simulink model "comparando_simulacoes_rate_diferente_entre_sensor_e_controlador"  (R2012b)
settings: Solver=ode3  StartTime=0.0  StopTime=1  FixedStep=1e-5  RelTol=1e-6
undefined symbols (not defined in the file): J, Kd, Ke, Kt, L, P, R
libraries: simulink x86
(part 1 of 3)
settings Model: BufferReuse=off  Creator=Juliano  LastModifiedBy=Juliano
settings OptimizationCC: OptimizeBlockIOStorage=off  BufferReuse=off  ExpressionFolding=off  LocalBlockOutputs=off

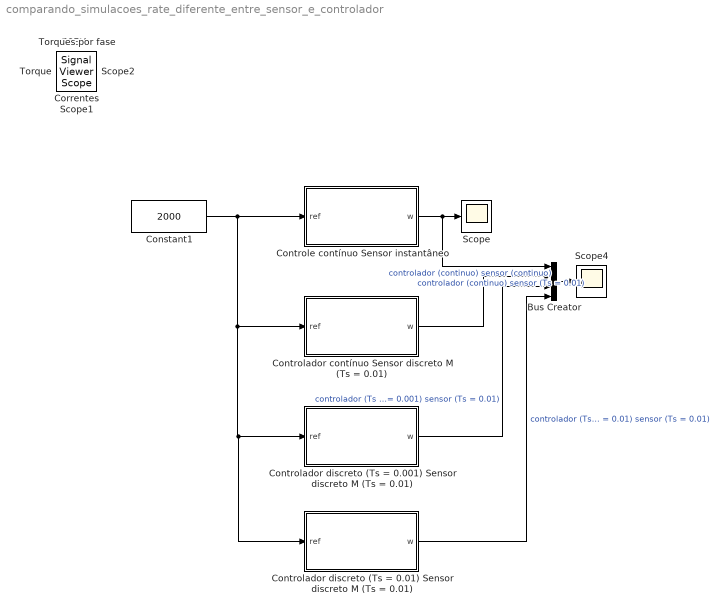
== system comparando_simulacoes_rate_diferente_entre_sensor_e_controlador ==
  Bus Creator : BusCreator
  Constant1 : Constant  Value=2000
  Controlador contínuo Sensor discreto M (Ts = 0.01) : Subsystem
  Controlador discreto (Ts = 0.001) Sensor discreto M (Ts = 0.01) : Subsystem
  Controlador discreto (Ts = 0.01) Sensor discreto M (Ts = 0.01) : Subsystem
  Controle contínuo Sensor instantâneo : Subsystem
  Scope : Scope
      settings: TimeRange=1  YMin=1600  YMax=3000
  Scope4 : Scope
      settings: ShowLegends=on  TimeRange=0.6  YMin=1100  YMax=3400  SaveName=ScopeData7
  Correntes : SignalViewerScope  IOType=viewer  NumInputPorts=3  ZoomMode=yonly  RefreshTime=0.035000
      settings: YMin=-5~-5~-5  YMax=5~5~5
  FCEMs : SignalViewerScope  IOType=viewer  NumInputPorts=3  RefreshTime=0.035000
      settings: YMin=-5~-5~-5  YMax=5~5~5  SaveName=ScopeData2
  Scope1 : SignalViewerScope  IOType=viewer  RefreshTime=0.035000
      settings: SaveName=ScopeData3
  Scope2 : SignalViewerScope  IOType=viewer  RefreshTime=0.035000
      settings: SaveName=ScopeData4
  Torque : SignalViewerScope  IOType=viewer  ZoomMode=xonly  RefreshTime=0.035000
      settings: SaveToWorkspace=on  SaveName=Torque
  Torques por fase : SignalViewerScope  IOType=viewer  NumInputPorts=3  ZoomMode=xonly  RefreshTime=0.035000
      settings: YMin=-5~-5~-5  YMax=5~5~5
  wires:
  Bus Creator/1 -> Scope4/1
  Controle contínuo Sensor instantâneo/1(w) -> Bus Creator/1, Scope/1  "controlador (continuo) sensor (continuo)"
  Constant1/1 -> Controlador contínuo Sensor discreto M (Ts = 0.01)/1(ref), Controlador discreto (Ts = 0.01) Sensor discreto M (Ts = 0.01)/1(ref), Controlador discreto (Ts = 0.001) Sensor discreto M (Ts = 0.01)/1(ref), Controle contínuo Sensor instantâneo/1(ref)
  Controlador discreto (Ts = 0.001) Sensor discreto M (Ts = 0.01)/1(w) -> Bus Creator/3  "controlador (Ts = 0.001) sensor (Ts = 0.01)"
  Controlador contínuo Sensor discreto M (Ts = 0.01)/1(w) -> Bus Creator/2  "controlador (continuo) sensor (Ts = 0.01)"
  Controlador discreto (Ts = 0.01) Sensor discreto M (Ts = 0.01)/1(w) -> Bus Creator/4  "controlador (Ts = 0.01) sensor (Ts = 0.01)"

== system comparando_simulacoes_rate_diferente_entre_sensor_e_controlador/Controlador contínuo Sensor discreto M (Ts = 0.01) ==
  ref : Inport
  Add2 : Sum  Inputs=-+|
  Anti-horário1 : Constant
  BLDC1 : Subsystem
  "Conversao deg/s -> rad/s" : Gain  Gain=pi/180
  Conversao rad-> deg : Gain  Gain=180/pi
  "Conversao rad/s -> RPM1" : Gain  Gain=60/(2*pi)
  "Conversao rad/s -> rpm" : Gain  Gain=60/(2*pi)
  Decoder1 : Subsystem
  Encoder : Subsystem  mask{Nr=360}
      mask prompts: Nr "Número de pulsos por revolução"
  Gain1 : Gain  Gain=P/2
  Inversor1 : Subsystem
  PID Controller1 : simulink/Continuous/PID Controller  Controller=PI  TimeDomain=Continuous-time  SampleTime=1  IntegratorMethod=Forward Euler  FilterMethod=Forward Euler  Form=Parallel  P=0.000518154594293452  I=0.0431725782178291  D=0  N=100  InitialConditionSource=internal  InitialConditionForIntegrator=0  InitialConditionForFilter=0  ExternalReset=none  ZeroCross=off  LimitOutput=on  UpperSaturationLimit=12  LowerSaturationLimit=-12  LinearizeAsGain=off  AntiWindupMode=none  Kb=1  TrackingMode=off  Kt=1  PParamMin=[ ]  PParamMax=[ ]  IParamMin=[ ]  IParamMax=[ ]  DParamMin=[ ]  DParamMax=[ ]  NParamMin=[ ]  NParamMax=[ ]  KbParamMin=[ ]  KbParamMax=[ ]  KtParamMin=[ ]  KtParamMax=[ ]  POutMin=[ ]  POutMax=[ ]  IOutMin=[ ]  IOutMax=[ ]  DOutMin=[ ]  DOutMax=[ ]  NOutMin=[ ]  NOutMax=[ ]  KbOutMin=[ ]  KbOutMax=[ ]  KtOutMin=[ ]  KtOutMax=[ ]  IntegratorOutMin=[ ]  IntegratorOutMax=[ ]  FilterOutMin=[ ]  FilterOutMax=[ ]  SumOutMin=[ ]  SumOutMax=[ ]  SumI1OutMin=[ ]  SumI1OutMax=[ ]  SumI2OutMin=[ ]  SumI2OutMax=[ ]  SumI3OutMin=[ ]  SumI3OutMax=[ ]  SumDOutMin=[ ]  SumDOutMax=[ ]  SaturationOutMin=[ ]  SaturationOutMax=[ ]  IntegratorContinuousStateAttributes=''  IntegratorStateMustResolveToSignalObject=off  IntegratorRTWStateStorageClass=Auto  FilterContinuousStateAttributes=''  FilterStateMustResolveToSignalObject=off  FilterRTWStateStorageClass=Auto
  Sensores Hall1 : Subsystem  AncestorBlock=spsPMSynchronousMachineModel/Discrete Trapezoidal/Hall effect sensor
  Step1 : Step  Time=0.2  After=0*2e-3  SampleTime=0
  w : Outport
  wires:
  Conversao rad-> deg/1 -> Encoder/1(Theta)
  "Conversao deg/s -> rad/s"/1 -> "Conversao rad/s -> rpm"/1
  ref/1 -> Add2/2
  PID Controller1/1 -> Inversor1/2(Vcc)
  "Conversao rad/s -> RPM1"/1 -> w/1
  Sensores Hall1/1(Hall) -> Decoder1/1("Hall ")
  Anti-horário1/1 -> Decoder1/2(Sentido de rotação)
  Inversor1/2(Vb) -> BLDC1/2(Vb)
  Add2/1 -> PID Controller1/1
  Inversor1/1(Va) -> BLDC1/1(Va)
  Decoder1/1(Gates) -> Inversor1/1(Gates)
  Inversor1/3(Vc) -> BLDC1/3(Vc)
  Gain1/1 -> Sensores Hall1/1(teta_e)
  BLDC1/1(Theta_m) -> Conversao rad-> deg/1, Gain1/1
  BLDC1/2(w_m) -> "Conversao rad/s -> RPM1"/1
  Step1/1 -> BLDC1/4(Tl)
  Encoder/3(VelocidadeM) -> "Conversao deg/s -> rad/s"/1
  "Conversao rad/s -> rpm"/1 -> Add2/1

== system comparando_simulacoes_rate_diferente_entre_sensor_e_controlador/Controlador discreto (Ts = 0.001) Sensor discreto M (Ts = 0.01) ==
  ref : Inport
  Add2 : Sum  Inputs=-+|
  Anti-horário1 : Constant
  BLDC1 : Subsystem
  "Conversao deg/s -> rad/s" : Gain  Gain=pi/180
  Conversao rad-> deg : Gain  Gain=180/pi
  "Conversao rad/s -> RPM1" : Gain  Gain=60/(2*pi)
  "Conversao rad/s -> rpm" : Gain  Gain=60/(2*pi)
  Decoder1 : Subsystem
  Discrete Transfer Fcn : DiscreteTransferFcn  Numerator=[-0.000518155 0.000474982]  Denominator=[-1 1]  SampleTime=0.001
  Encoder : Subsystem  mask{Nr=360}
      mask prompts: Nr "Número de pulsos por revolução"
  Gain1 : Gain  Gain=P/2
  Inversor1 : Subsystem
  Rate Transition : RateTransition  OutPortSampleTimeOpt=Inherit
  Rate Transition1 : RateTransition  OutPortSampleTimeOpt=Inherit
  Saturation : Saturate  UpperLimit=12  LowerLimit=-12
  Sensores Hall1 : Subsystem  AncestorBlock=spsPMSynchronousMachineModel/Discrete Trapezoidal/Hall effect sensor
  Step1 : Step  Time=0.2  After=0*2e-3  SampleTime=0
  w : Outport
  wires:
  "Conversao rad/s -> rpm"/1 -> Add2/1
  Encoder/3(VelocidadeM) -> "Conversao deg/s -> rad/s"/1
  Step1/1 -> BLDC1/4(Tl)
  BLDC1/2(w_m) -> "Conversao rad/s -> RPM1"/1
  BLDC1/1(Theta_m) -> Gain1/1, Conversao rad-> deg/1
  Gain1/1 -> Sensores Hall1/1(teta_e)
  Inversor1/3(Vc) -> BLDC1/3(Vc)
  Decoder1/1(Gates) -> Inversor1/1(Gates)
  Inversor1/1(Va) -> BLDC1/1(Va)
  Inversor1/2(Vb) -> BLDC1/2(Vb)
  Anti-horário1/1 -> Decoder1/2(Sentido de rotação)
  Sensores Hall1/1(Hall) -> Decoder1/1("Hall ")
  "Conversao rad/s -> RPM1"/1 -> w/1
  ref/1 -> Add2/2
  "Conversao deg/s -> rad/s"/1 -> "Conversao rad/s -> rpm"/1
  Conversao rad-> deg/1 -> Encoder/1(Theta)
  Add2/1 -> Rate Transition/1
  Rate Transition1/1 -> Inversor1/2(Vcc)
  Discrete Transfer Fcn/1 -> Saturation/1
  Rate Transition/1 -> Discrete Transfer Fcn/1
  Saturation/1 -> Rate Transition1/1

== system comparando_simulacoes_rate_diferente_entre_sensor_e_controlador/Controlador discreto (Ts = 0.01) Sensor discreto M (Ts = 0.01) ==
  ref : Inport
  Add2 : Sum  Inputs=-+|
  Anti-horário1 : Constant
  BLDC1 : Subsystem
  "Conversao deg/s -> rad/s" : Gain  Gain=pi/180
  Conversao rad-> deg : Gain  Gain=180/pi
  "Conversao rad/s -> RPM1" : Gain  Gain=60/(2*pi)
  "Conversao rad/s -> rpm" : Gain  Gain=60/(2*pi)
  Decoder1 : Subsystem
  Discrete Transfer Fcn : DiscreteTransferFcn  Numerator=[-0.000518155 0.0000864288]  Denominator=[-1 1]  SampleTime=0.01
  Encoder : Subsystem  mask{Nr=360}
      mask prompts: Nr "Número de pulsos por revolução"
  Gain1 : Gain  Gain=P/2
  Inversor1 : Subsystem
  Rate Transition : RateTransition  OutPortSampleTimeOpt=Inherit
  Rate Transition1 : RateTransition  OutPortSampleTimeOpt=Inherit
  Saturation : Saturate  UpperLimit=12  LowerLimit=-12
  Sensores Hall1 : Subsystem  AncestorBlock=spsPMSynchronousMachineModel/Discrete Trapezoidal/Hall effect sensor
  Step1 : Step  Time=0.2  After=0*2e-3  SampleTime=0
  w : Outport
  wires:
  Saturation/1 -> Rate Transition1/1
  Rate Transition/1 -> Discrete Transfer Fcn/1
  Discrete Transfer Fcn/1 -> Saturation/1
  Rate Transition1/1 -> Inversor1/2(Vcc)
  Add2/1 -> Rate Transition/1
  Conversao rad-> deg/1 -> Encoder/1(Theta)
  "Conversao deg/s -> rad/s"/1 -> "Conversao rad/s -> rpm"/1
  ref/1 -> Add2/2
  "Conversao rad/s -> RPM1"/1 -> w/1
  Sensores Hall1/1(Hall) -> Decoder1/1("Hall ")
  Anti-horário1/1 -> Decoder1/2(Sentido de rotação)
  Inversor1/2(Vb) -> BLDC1/2(Vb)
  Inversor1/1(Va) -> BLDC1/1(Va)
  Decoder1/1(Gates) -> Inversor1/1(Gates)
  Inversor1/3(Vc) -> BLDC1/3(Vc)
  Gain1/1 -> Sensores Hall1/1(teta_e)
  BLDC1/1(Theta_m) -> Conversao rad-> deg/1, Gain1/1
  BLDC1/2(w_m) -> "Conversao rad/s -> RPM1"/1
  Step1/1 -> BLDC1/4(Tl)
  Encoder/3(VelocidadeM) -> "Conversao deg/s -> rad/s"/1
  "Conversao rad/s -> rpm"/1 -> Add2/1

== system comparando_simulacoes_rate_diferente_entre_sensor_e_controlador/Controle contínuo Sensor instantâneo ==
  ref : Inport
  Add1 : Sum  Inputs=|+-
  Anti-horário : Constant
  BLDC : Subsystem
  "Conversao rad/s -> RPM" : Gain  Gain=60/(2*pi)
  Decoder : Subsystem
  Gain : Gain  Gain=P/2
  Inversor : Subsystem
  PID Controller : simulink/Continuous/PID Controller  Controller=PI  TimeDomain=Continuous-time  SampleTime=1  IntegratorMethod=Forward Euler  FilterMethod=Forward Euler  Form=Parallel  P=0.000518154594293452  I=0.0431725782178291  D=0  N=100  InitialConditionSource=internal  InitialConditionForIntegrator=0  InitialConditionForFilter=0  ExternalReset=none  ZeroCross=off  LimitOutput=on  UpperSaturationLimit=12  LowerSaturationLimit=-12  LinearizeAsGain=off  AntiWindupMode=none  Kb=1  TrackingMode=off  Kt=1  PParamMin=[ ]  PParamMax=[ ]  IParamMin=[ ]  IParamMax=[ ]  DParamMin=[ ]  DParamMax=[ ]  NParamMin=[ ]  NParamMax=[ ]  KbParamMin=[ ]  KbParamMax=[ ]  KtParamMin=[ ]  KtParamMax=[ ]  POutMin=[ ]  POutMax=[ ]  IOutMin=[ ]  IOutMax=[ ]  DOutMin=[ ]  DOutMax=[ ]  NOutMin=[ ]  NOutMax=[ ]  KbOutMin=[ ]  KbOutMax=[ ]  KtOutMin=[ ]  KtOutMax=[ ]  IntegratorOutMin=[ ]  IntegratorOutMax=[ ]  FilterOutMin=[ ]  FilterOutMax=[ ]  SumOutMin=[ ]  SumOutMax=[ ]  SumI1OutMin=[ ]  SumI1OutMax=[ ]  SumI2OutMin=[ ]  SumI2OutMax=[ ]  SumI3OutMin=[ ]  SumI3OutMax=[ ]  SumDOutMin=[ ]  SumDOutMax=[ ]  SaturationOutMin=[ ]  SaturationOutMax=[ ]  IntegratorContinuousStateAttributes=''  IntegratorStateMustResolveToSignalObject=off  IntegratorRTWStateStorageClass=Auto  FilterContinuousStateAttributes=''  FilterStateMustResolveToSignalObject=off  FilterRTWStateStorageClass=Auto
  Sensores Hall : Subsystem  AncestorBlock=spsPMSynchronousMachineModel/Discrete Trapezoidal/Hall effect sensor
  Step : Step  Time=0.2  After=0*2e-3  SampleTime=0
  w : Outport
  wires:
  PID Controller/1 -> Inversor/2(Vcc)
  BLDC/1(Theta_m) -> Gain/1
  Gain/1 -> Sensores Hall/1(teta_e)
  Sensores Hall/1(Hall) -> Decoder/1("Hall ")
  Decoder/1(Gates) -> Inversor/1(Gates)
  Anti-horário/1 -> Decoder/2(Sentido de rotação)
  Step/1 -> BLDC/4(Tl)
  Inversor/1(Va) -> BLDC/1(Va)
  Inversor/2(Vb) -> BLDC/2(Vb)
  Inversor/3(Vc) -> BLDC/3(Vc)
  BLDC/2(w_m) -> "Conversao rad/s -> RPM"/1
  "Conversao rad/s -> RPM"/1 -> w/1, Add1/2
  Add1/1 -> PID Controller/1
  ref/1 -> Add1/1

== system comparando_simulacoes_rate_diferente_entre_sensor_e_controlador/Controlador contínuo Sensor discreto M (Ts = 0.01)/BLDC1 ==
  Va : Inport
  Vb : Inport  Port=2
  Vc : Inport  Port=3
  Tl : Inport  Port=4
  "Cálculo Torque fase \"a\"" : Subsystem
  "Cálculo Torque fase \"b\"" : Subsystem
  "Cálculo Torque fase \"c\"" : Subsystem
  Cálculo das FCEMs : Subsystem
  "Dinâmica fase \"a\"" : Subsystem
  "Dinâmica fase \"b\"" : Subsystem
  "Dinâmica fase \"c\"" : Subsystem
  "Dinâmica mecânica " : Subsystem
  FCEMs : Scope  NumInputPorts=3
      settings: TimeRange=1  YMin=420~-5~-5  YMax=510~5~5  SaveName=ScopeData5
  Gain2 : Gain  Gain=P/2
  Scope : Scope
      settings: TimeRange=1  YMin=420  YMax=510  SaveName=ScopeData4
  Sum : Sum  Inputs=+++
  Vs : Scope  NumInputPorts=3
      settings: TimeRange=1  YMin=420~-5~-5  YMax=510~5~5  SaveName=ScopeData2
  is : Scope  NumInputPorts=3
      settings: TimeRange=1  YMin=420~-5~-5  YMax=510~5~5  SaveName=ScopeData3
  is1 : Scope  NumInputPorts=3
      settings: TimeRange=1  YMin=420~-5~-5  YMax=510~5~5  SaveName=ScopeData6
  Theta_m : Outport
  w_m : Outport  Port=2
  wires:
  Cálculo das FCEMs/1(e_a) -> FCEMs/1, "Dinâmica fase \"a\""/2(e_a)  "e_a"
  Cálculo das FCEMs/2(e_b) -> "Dinâmica fase \"b\""/2(e_b), FCEMs/2  "e_b"
  Cálculo das FCEMs/3(e_c) -> FCEMs/3, "Dinâmica fase \"c\""/2(e_c)  "e_c"
  Va/1 -> Vs/1, "Dinâmica fase \"a\""/1(Va)
  Vb/1 -> Vs/2, "Dinâmica fase \"b\""/1(Vb)
  Vc/1 -> Vs/3, "Dinâmica fase \"c\""/1(Vc)
  "Dinâmica fase \"a\""/1(i_a) -> is/1, "Cálculo Torque fase \"a\""/1(i_a)  "i_a"
  "Dinâmica fase \"b\""/1(i_b) -> is/2, "Cálculo Torque fase \"b\""/1(i_b)  "i_b"
  "Dinâmica fase \"c\""/1(i_c) -> is/3, "Cálculo Torque fase \"c\""/1(i_c)  "i_c"
  "Cálculo Torque fase \"a\""/1(T_a) -> is1/1, Sum/1  "T_a"
  "Cálculo Torque fase \"b\""/1(T_b) -> is1/2, Sum/2  "T_b"
  "Cálculo Torque fase \"c\""/1(T_c) -> is1/3, Sum/3  "T_c"
  Sum/1 -> Scope/1, "Dinâmica mecânica "/1(Te)  "T"
  "Dinâmica mecânica "/1(Theta_m) -> Theta_m/1, Gain2/1  "Theta_m"
  "Dinâmica mecânica "/2(w_m) -> Cálculo das FCEMs/2(w_m), w_m/1  "w_m"
  Tl/1 -> "Dinâmica mecânica "/2(Tl)
  Gain2/1 -> "Cálculo Torque fase \"a\""/2(Theta_e), "Cálculo Torque fase \"c\""/2(Theta_e), Cálculo das FCEMs/1(Theta_e), "Cálculo Torque fase \"b\""/2(Theta_e)

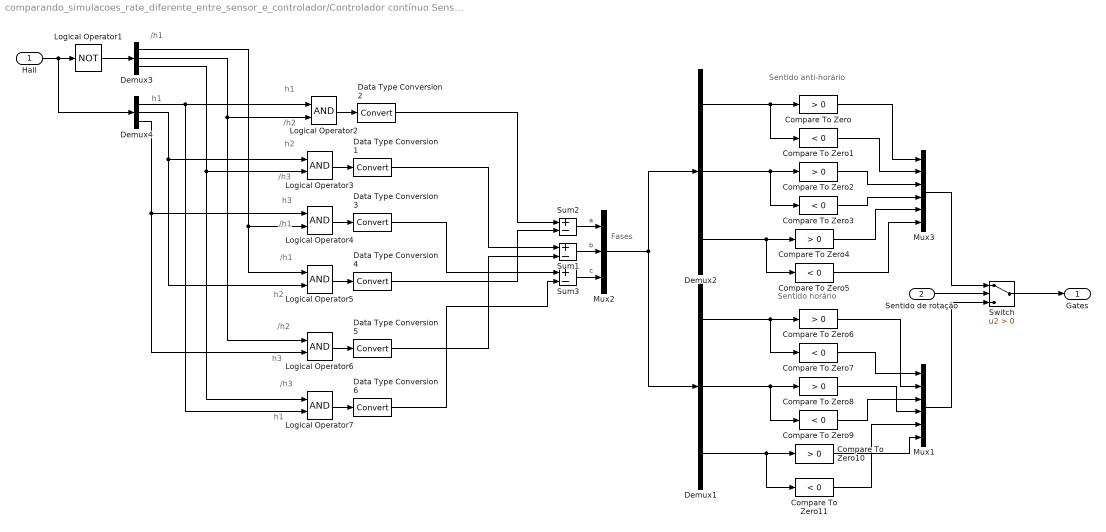
== system comparando_simulacoes_rate_diferente_entre_sensor_e_controlador/Controlador contínuo Sensor discreto M (Ts = 0.01)/Decoder1 ==
  note: Fases
  note: Sentido horário
  note: Sentido anti-horário
  note: h1
  note: /h3
  note: h3
  note: /h2
  note: h2
  note: /h1
  note: /h1
  note: h3
  note: /h3
  note: h2
  note: /h2
  note: h1
  note: h1
  note: /h1
  "Hall " : Inport
  Sentido de rotação : Inport  Port=2
  Compare To Zero{,2,4,6,8,10} (6 alike) : simulink/Logic and Bit Operations/Compare To Zero  relop=>  OutDataTypeStr=boolean  ZeroCross=off
  Compare To Zero{1,3,5,7,9,11} (6 alike) : simulink/Logic and Bit Operations/Compare To Zero  relop=<  OutDataTypeStr=boolean  ZeroCross=off
  Data Type Conversion{1..6} (6 alike) : DataTypeConversion
  Demux{1..4} (4 alike) : Demux  Outputs=3
  Logical Operator1 : Logic  Operator=NOT  AllPortsSameDT=off  OutDataTypeStr=boolean
  Logical Operator{2..7} (6 alike) : Logic  AllPortsSameDT=off  OutDataTypeStr=boolean
  Mux1 : Mux  Inputs=6
  Mux2 : Mux  Inputs=3
  Mux3 : Mux  Inputs=6
  Sum1 : Sum  Inputs=+-  OutDataTypeStr=double
  Sum2 : Sum  Inputs=+-  OutDataTypeStr=double
  Sum3 : Sum  Inputs=+-  OutDataTypeStr=double
  Switch : Switch  Criteria=u2 > Threshold
  Gates : Outport
  wires:
  Mux2/1 -> Demux1/1, Demux2/1
  Data Type Conversion6/1 -> Sum3/2
  Data Type Conversion3/1 -> Sum3/1
  Data Type Conversion5/1 -> Sum1/2
  Data Type Conversion1/1 -> Sum1/1
  Data Type Conversion4/1 -> Sum2/2
  Data Type Conversion2/1 -> Sum2/1
  Logical Operator7/1 -> Data Type Conversion6/1
  Logical Operator6/1 -> Data Type Conversion5/1
  Logical Operator5/1 -> Data Type Conversion4/1
  Logical Operator4/1 -> Data Type Conversion3/1
  Logical Operator3/1 -> Data Type Conversion1/1
  Sum3/1 -> Mux2/3  "c"
  Sum1/1 -> Mux2/2  "b"
  Sum2/1 -> Mux2/1  "a"
  Logical Operator2/1 -> Data Type Conversion2/1
  Demux3/1 -> Logical Operator5/1, Logical Operator4/2
  Demux3/2 -> Logical Operator6/1, Logical Operator2/2
  Demux3/3 -> Logical Operator7/1, Logical Operator3/2
  Demux4/1 -> Logical Operator7/2, Logical Operator2/1
  Demux4/2 -> Logical Operator5/2, Logical Operator3/1
  Demux4/3 -> Logical Operator6/2, Logical Operator4/1
  Logical Operator1/1 -> Demux3/1
  "Hall "/1 -> Demux4/1, Logical Operator1/1
  Compare To Zero10/1 -> Mux1/6
  Compare To Zero11/1 -> Mux1/5
  Compare To Zero8/1 -> Mux1/4
  Compare To Zero9/1 -> Mux1/3
  Compare To Zero6/1 -> Mux1/2
  Compare To Zero7/1 -> Mux1/1
  Switch/1 -> Gates/1
  Mux1/1 -> Switch/3
  Sentido de rotação/1 -> Switch/2
  Mux3/1 -> Switch/1
  Demux1/3 -> Compare To Zero11/1, Compare To Zero10/1
  Demux1/2 -> Compare To Zero9/1, Compare To Zero8/1
  Demux1/1 -> Compare To Zero7/1, Compare To Zero6/1
  Compare To Zero5/1 -> Mux3/6
  Compare To Zero4/1 -> Mux3/5
  Compare To Zero3/1 -> Mux3/4
  Compare To Zero2/1 -> Mux3/3
  Compare To Zero1/1 -> Mux3/2
  Compare To Zero/1 -> Mux3/1
  Demux2/3 -> Compare To Zero5/1, Compare To Zero4/1
  Demux2/2 -> Compare To Zero3/1, Compare To Zero2/1
  Demux2/1 -> Compare To Zero1/1, Compare To Zero/1

== system comparando_simulacoes_rate_diferente_entre_sensor_e_controlador/Controlador contínuo Sensor discreto M (Ts = 0.01)/Encoder ==
  note: ATENÇÃO: Para o correto funcionamento desse encoder o step size da simulação deve ser menor do que 360/(4*Nr*Vmax),
      | onde Vmax é o valor máximo da derivada do Theta atigindo durante a simulação
  Theta : Inport
  Determinar direçao : Subsystem
  Graus / pulso1 : Gain  Gain=360/(4*Nr)  OutDataTypeStr=double
  Método M : Subsystem  mask{Ts=0.01}
      mask prompts: Ts "Sampling time"
  Método T : Subsystem  mask{m=1}
      mask prompts: m "Número de pulsos que o bloco espera para calcular a velocidade média"
  Sensor Óptico : Subsystem
  Sensor Óptico1 : Subsystem
  Subsystem : Subsystem
  Theta_amostrado : Outport
  VelocidadeT : Outport  Port=2
  VelocidadeM : Outport  Port=3
  wires:
  Método M/1(Velocidade) -> VelocidadeM/1
  Método T/1(Velocidade) -> VelocidadeT/1
  Theta/1 -> Sensor Óptico/1(Theta), Sensor Óptico1/1(Theta)
  Graus / pulso1/1 -> Theta_amostrado/1, Método M/1(Posição)
  Subsystem/1(Out) -> Graus / pulso1/1
  Determinar direçao/2(NEG) -> Subsystem/2(NEG)
  Determinar direçao/1(POS) -> Subsystem/1(POS)
  Sensor Óptico1/1(Sinal_Pulso) -> Determinar direçao/2(B), Método T/2(B)  "B"
  Sensor Óptico/1(Sinal_Pulso) -> Método T/1(A), Determinar direçao/1(A)  "A"

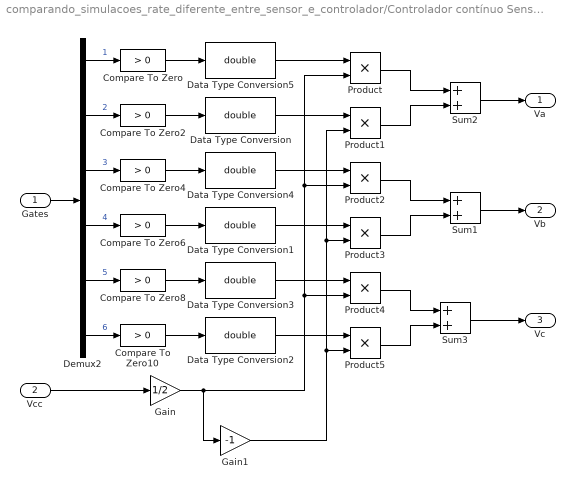
== system comparando_simulacoes_rate_diferente_entre_sensor_e_controlador/Controlador contínuo Sensor discreto M (Ts = 0.01)/Inversor1 ==
  Gates : Inport
  Vcc : Inport  Port=2
  Compare To Zero : simulink/Logic and Bit Operations/Compare To Zero  relop=>  OutDataTypeStr=uint8  ZeroCross=off
  Compare To Zero{2,6,8,10} (4 alike) : simulink/Logic and Bit Operations/Compare To Zero  relop=>  OutDataTypeStr=boolean  ZeroCross=off
  Compare To Zero4 : simulink/Logic and Bit Operations/Compare To Zero  relop=>  OutDataTypeStr=uint8  ZeroCross=off
  Data Type Conversion{,1..5} (6 alike) : DataTypeConversion  OutDataTypeStr=double
  Demux2 : Demux  Outputs=6
  Gain : Gain  Gain=1/2
  Gain1 : Gain  Gain=-1
  Product{,1..5} (6 alike) : Product  RndMeth=Zero
  Sum1 : Sum  SaturateOnIntegerOverflow=on
  Sum2 : Sum  SaturateOnIntegerOverflow=on
  Sum3 : Sum  SaturateOnIntegerOverflow=on
  Va : Outport
  Vb : Outport  Port=2
  Vc : Outport  Port=3
  wires:
  Vcc/1 -> Gain/1
  Sum1/1 -> Vb/1
  Sum3/1 -> Vc/1
  Sum2/1 -> Va/1
  Gates/1 -> Demux2/1
  Demux2/1 -> Compare To Zero/1  "1"
  Demux2/2 -> Compare To Zero2/1  "2"
  Demux2/3 -> Compare To Zero4/1  "3"
  Demux2/4 -> Compare To Zero6/1  "4"
  Demux2/5 -> Compare To Zero8/1  "5"
  Demux2/6 -> Compare To Zero10/1  "6"
  Compare To Zero/1 -> Data Type Conversion5/1
  Compare To Zero2/1 -> Data Type Conversion/1
  Compare To Zero4/1 -> Data Type Conversion4/1
  Compare To Zero6/1 -> Data Type Conversion1/1
  Compare To Zero8/1 -> Data Type Conversion3/1
  Compare To Zero10/1 -> Data Type Conversion2/1
  Product/1 -> Sum2/1
  Product1/1 -> Sum2/2
  Product2/1 -> Sum1/1
  Product3/1 -> Sum1/2
  Product4/1 -> Sum3/1
  Product5/1 -> Sum3/2
  Data Type Conversion2/1 -> Product5/1
  Data Type Conversion3/1 -> Product4/1
  Data Type Conversion1/1 -> Product3/1
  Data Type Conversion4/1 -> Product2/1
  Data Type Conversion/1 -> Product1/1
  Data Type Conversion5/1 -> Product/1
  Gain1/1 -> Product5/2, Product3/2, Product1/2
  Gain/1 -> Gain1/1, Product4/2, Product2/2, Product/2

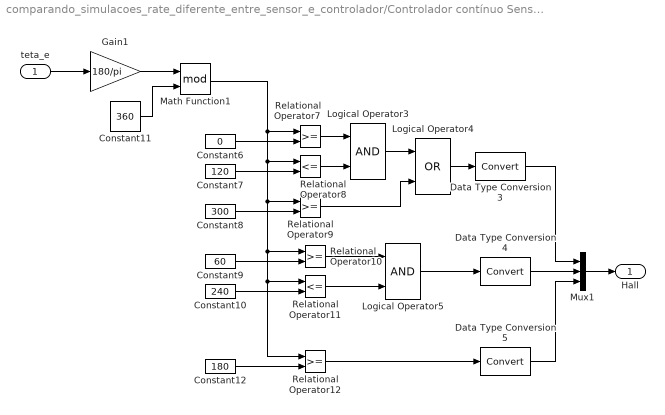
== system comparando_simulacoes_rate_diferente_entre_sensor_e_controlador/Controlador contínuo Sensor discreto M (Ts = 0.01)/Sensores Hall1 ==
  teta_e : Inport
  Constant10 : Constant  Value=240
  Constant11 : Constant  Value=360
  Constant12 : Constant  Value=180
  Constant6 : Constant  Value=0
  Constant7 : Constant  Value=120
  Constant8 : Constant  Value=300
  Constant9 : Constant  Value=60
  Data Type Conversion3 : DataTypeConversion  SaturateOnIntegerOverflow=on  RndMeth=Zero
  Data Type Conversion4 : DataTypeConversion  SaturateOnIntegerOverflow=on  RndMeth=Zero
  Data Type Conversion5 : DataTypeConversion  SaturateOnIntegerOverflow=on  RndMeth=Zero
  Gain1 : Gain  Gain=180/pi
  Logical Operator3 : Logic  AllPortsSameDT=off  OutDataTypeStr=boolean
  Logical Operator4 : Logic  Operator=OR  AllPortsSameDT=off  OutDataTypeStr=boolean
  Logical Operator5 : Logic  AllPortsSameDT=off  OutDataTypeStr=boolean
  Math Function1 : Math  Operator=mod  SaturateOnIntegerOverflow=on
  Mux1 : Mux  Inputs=3
  Relational Operator{7,9..10,12} (4 alike) : RelationalOperator  InputSameDT=on
  Relational Operator11 : RelationalOperator  Operator=<=  InputSameDT=on
  Relational Operator8 : RelationalOperator  Operator=<=  InputSameDT=on
  Hall : Outport
  wires:
  teta_e/1 -> Gain1/1
  Constant6/1 -> Relational Operator7/2
  Constant7/1 -> Relational Operator8/2
  Constant8/1 -> Relational Operator9/2
  Relational Operator9/1 -> Logical Operator4/2
  Logical Operator3/1 -> Logical Operator4/1
  Relational Operator7/1 -> Logical Operator3/1
  Relational Operator8/1 -> Logical Operator3/2
  Relational Operator10/1 -> Logical Operator5/1
  Relational Operator11/1 -> Logical Operator5/2
  Constant9/1 -> Relational Operator10/2
  Constant10/1 -> Relational Operator11/2
  Constant12/1 -> Relational Operator12/2
  Mux1/1 -> Hall/1
  Data Type Conversion3/1 -> Mux1/1
  Data Type Conversion4/1 -> Mux1/2
  Data Type Conversion5/1 -> Mux1/3
  Logical Operator4/1 -> Data Type Conversion3/1
  Logical Operator5/1 -> Data Type Conversion4/1
  Relational Operator12/1 -> Data Type Conversion5/1
  Gain1/1 -> Math Function1/1
  Constant11/1 -> Math Function1/2
  Math Function1/1 -> Relational Operator8/1, Relational Operator9/1, Relational Operator10/1, Relational Operator11/1, Relational Operator12/1, Relational Operator7/1

== system comparando_simulacoes_rate_diferente_entre_sensor_e_controlador/Controlador discreto (Ts = 0.001) Sensor discreto M (Ts = 0.01)/BLDC1 ==
  Va : Inport
  Vb : Inport  Port=2
  Vc : Inport  Port=3
  Tl : Inport  Port=4
  "Cálculo Torque fase \"a\"" : Subsystem
  "Cálculo Torque fase \"b\"" : Subsystem
  "Cálculo Torque fase \"c\"" : Subsystem
  Cálculo das FCEMs : Subsystem
  "Dinâmica fase \"a\"" : Subsystem
  "Dinâmica fase \"b\"" : Subsystem
  "Dinâmica fase \"c\"" : Subsystem
  "Dinâmica mecânica " : Subsystem
  FCEMs : Scope  NumInputPorts=3
      settings: TimeRange=1  YMin=420~-5~-5  YMax=510~5~5  SaveName=ScopeData5
  Gain2 : Gain  Gain=P/2
  Scope : Scope
      settings: TimeRange=1  YMin=420  YMax=510  SaveName=ScopeData4
  Sum : Sum  Inputs=+++
  Vs : Scope  NumInputPorts=3
      settings: TimeRange=1  YMin=420~-5~-5  YMax=510~5~5  SaveName=ScopeData2
  is : Scope  NumInputPorts=3
      settings: TimeRange=1  YMin=420~-5~-5  YMax=510~5~5  SaveName=ScopeData3
  is1 : Scope  NumInputPorts=3
      settings: TimeRange=1  YMin=420~-5~-5  YMax=510~5~5  SaveName=ScopeData6
  Theta_m : Outport
  w_m : Outport  Port=2
  wires:
  Gain2/1 -> "Cálculo Torque fase \"b\""/2(Theta_e), Cálculo das FCEMs/1(Theta_e), "Cálculo Torque fase \"c\""/2(Theta_e), "Cálculo Torque fase \"a\""/2(Theta_e)
  Tl/1 -> "Dinâmica mecânica "/2(Tl)
  "Dinâmica mecânica "/2(w_m) -> w_m/1, Cálculo das FCEMs/2(w_m)  "w_m"
  "Dinâmica mecânica "/1(Theta_m) -> Gain2/1, Theta_m/1  "Theta_m"
  Sum/1 -> "Dinâmica mecânica "/1(Te), Scope/1  "T"
  "Cálculo Torque fase \"c\""/1(T_c) -> Sum/3, is1/3  "T_c"
  "Cálculo Torque fase \"b\""/1(T_b) -> Sum/2, is1/2  "T_b"
  "Cálculo Torque fase \"a\""/1(T_a) -> Sum/1, is1/1  "T_a"
  "Dinâmica fase \"c\""/1(i_c) -> "Cálculo Torque fase \"c\""/1(i_c), is/3  "i_c"
  "Dinâmica fase \"b\""/1(i_b) -> "Cálculo Torque fase \"b\""/1(i_b), is/2  "i_b"
  "Dinâmica fase \"a\""/1(i_a) -> "Cálculo Torque fase \"a\""/1(i_a), is/1  "i_a"
  Vc/1 -> "Dinâmica fase \"c\""/1(Vc), Vs/3
  Vb/1 -> "Dinâmica fase \"b\""/1(Vb), Vs/2
  Va/1 -> "Dinâmica fase \"a\""/1(Va), Vs/1
  Cálculo das FCEMs/3(e_c) -> "Dinâmica fase \"c\""/2(e_c), FCEMs/3  "e_c"
  Cálculo das FCEMs/2(e_b) -> FCEMs/2, "Dinâmica fase \"b\""/2(e_b)  "e_b"
  Cálculo das FCEMs/1(e_a) -> "Dinâmica fase \"a\""/2(e_a), FCEMs/1  "e_a"

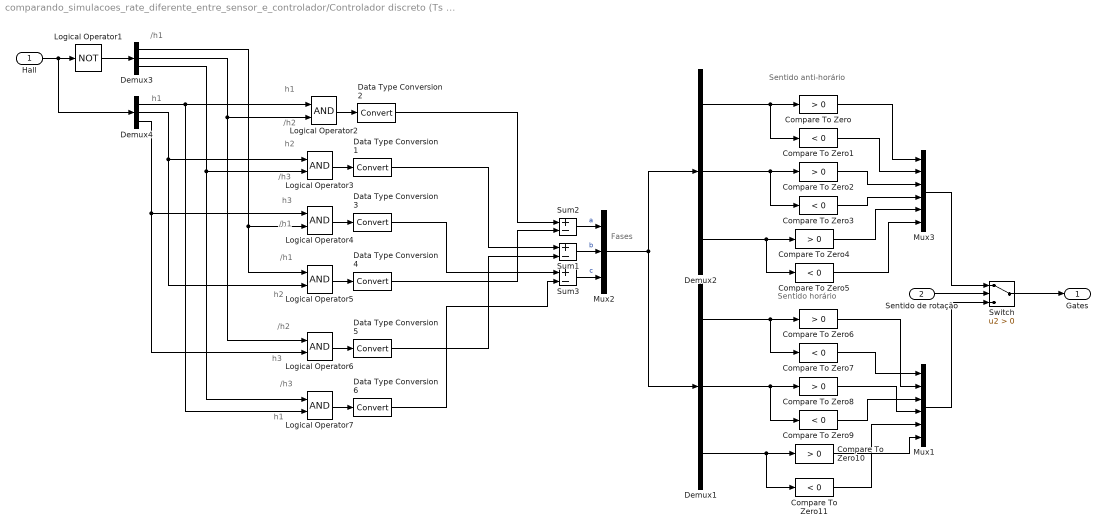
== system comparando_simulacoes_rate_diferente_entre_sensor_e_controlador/Controlador discreto (Ts = 0.001) Sensor discreto M (Ts = 0.01)/Decoder1 ==
  note: /h1
  note: h1
  note: h1
  note: /h2
  note: h2
  note: /h3
  note: h3
  note: /h1
  note: /h1
  note: h2
  note: /h2
  note: h3
  note: /h3
  note: h1
  note: Sentido anti-horário
  note: Sentido horário
  note: Fases
  "Hall " : Inport
  Sentido de rotação : Inport  Port=2
  Compare To Zero{,2,4,6,8,10} (6 alike) : simulink/Logic and Bit Operations/Compare To Zero  relop=>  OutDataTypeStr=boolean  ZeroCross=off
  Compare To Zero{1,3,5,7,9,11} (6 alike) : simulink/Logic and Bit Operations/Compare To Zero  relop=<  OutDataTypeStr=boolean  ZeroCross=off
  Data Type Conversion{1..6} (6 alike) : DataTypeConversion
  Demux{1..4} (4 alike) : Demux  Outputs=3
  Logical Operator1 : Logic  Operator=NOT  AllPortsSameDT=off  OutDataTypeStr=boolean
  Logical Operator{2..7} (6 alike) : Logic  AllPortsSameDT=off  OutDataTypeStr=boolean
  Mux1 : Mux  Inputs=6
  Mux2 : Mux  Inputs=3
  Mux3 : Mux  Inputs=6
  Sum1 : Sum  Inputs=+-  OutDataTypeStr=double
  Sum2 : Sum  Inputs=+-  OutDataTypeStr=double
  Sum3 : Sum  Inputs=+-  OutDataTypeStr=double
  Switch : Switch  Criteria=u2 > Threshold
  Gates : Outport
  wires:
  Demux2/1 -> Compare To Zero/1, Compare To Zero1/1
  Demux2/2 -> Compare To Zero2/1, Compare To Zero3/1
  Demux2/3 -> Compare To Zero4/1, Compare To Zero5/1
  Compare To Zero/1 -> Mux3/1
  Compare To Zero1/1 -> Mux3/2
  Compare To Zero2/1 -> Mux3/3
  Compare To Zero3/1 -> Mux3/4
  Compare To Zero4/1 -> Mux3/5
  Compare To Zero5/1 -> Mux3/6
  Demux1/1 -> Compare To Zero6/1, Compare To Zero7/1
  Demux1/2 -> Compare To Zero8/1, Compare To Zero9/1
  Demux1/3 -> Compare To Zero10/1, Compare To Zero11/1
  Mux3/1 -> Switch/1
  Sentido de rotação/1 -> Switch/2
  Mux1/1 -> Switch/3
  Switch/1 -> Gates/1
  Compare To Zero7/1 -> Mux1/1
  Compare To Zero6/1 -> Mux1/2
  Compare To Zero9/1 -> Mux1/3
  Compare To Zero8/1 -> Mux1/4
  Compare To Zero11/1 -> Mux1/5
  Compare To Zero10/1 -> Mux1/6
  "Hall "/1 -> Logical Operator1/1, Demux4/1
  Logical Operator1/1 -> Demux3/1
  Demux4/3 -> Logical Operator4/1, Logical Operator6/2
  Demux4/2 -> Logical Operator3/1, Logical Operator5/2
  Demux4/1 -> Logical Operator2/1, Logical Operator7/2
  Demux3/3 -> Logical Operator3/2, Logical Operator7/1
  Demux3/2 -> Logical Operator2/2, Logical Operator6/1
  Demux3/1 -> Logical Operator4/2, Logical Operator5/1
  Logical Operator2/1 -> Data Type Conversion2/1
  Sum2/1 -> Mux2/1  "a"
  Sum1/1 -> Mux2/2  "b"
  Sum3/1 -> Mux2/3  "c"
  Logical Operator3/1 -> Data Type Conversion1/1
  Logical Operator4/1 -> Data Type Conversion3/1
  Logical Operator5/1 -> Data Type Conversion4/1
  Logical Operator6/1 -> Data Type Conversion5/1
  Logical Operator7/1 -> Data Type Conversion6/1
  Data Type Conversion2/1 -> Sum2/1
  Data Type Conversion4/1 -> Sum2/2
  Data Type Conversion1/1 -> Sum1/1
  Data Type Conversion5/1 -> Sum1/2
  Data Type Conversion3/1 -> Sum3/1
  Data Type Conversion6/1 -> Sum3/2
  Mux2/1 -> Demux2/1, Demux1/1

== system comparando_simulacoes_rate_diferente_entre_sensor_e_controlador/Controlador discreto (Ts = 0.001) Sensor discreto M (Ts = 0.01)/Encoder ==
  note: ATENÇÃO: Para o correto funcionamento desse encoder o step size da simulação deve ser menor do que 360/(4*Nr*Vmax),
      | onde Vmax é o valor máximo da derivada do Theta atigindo durante a simulação
  Theta : Inport
  Determinar direçao : Subsystem
  Graus / pulso1 : Gain  Gain=360/(4*Nr)  OutDataTypeStr=double
  Método M : Subsystem  mask{Ts=0.01}
      mask prompts: Ts "Sampling time"
  Método T : Subsystem  mask{m=1}
      mask prompts: m "Número de pulsos que o bloco espera para calcular a velocidade média"
  Sensor Óptico : Subsystem
  Sensor Óptico1 : Subsystem
  Subsystem : Subsystem
  Theta_amostrado : Outport
  VelocidadeT : Outport  Port=2
  VelocidadeM : Outport  Port=3
  wires:
  Sensor Óptico/1(Sinal_Pulso) -> Determinar direçao/1(A), Método T/1(A)  "A"
  Sensor Óptico1/1(Sinal_Pulso) -> Método T/2(B), Determinar direçao/2(B)  "B"
  Determinar direçao/1(POS) -> Subsystem/1(POS)
  Determinar direçao/2(NEG) -> Subsystem/2(NEG)
  Subsystem/1(Out) -> Graus / pulso1/1
  Graus / pulso1/1 -> Método M/1(Posição), Theta_amostrado/1
  Theta/1 -> Sensor Óptico1/1(Theta), Sensor Óptico/1(Theta)
  Método T/1(Velocidade) -> VelocidadeT/1
  Método M/1(Velocidade) -> VelocidadeM/1

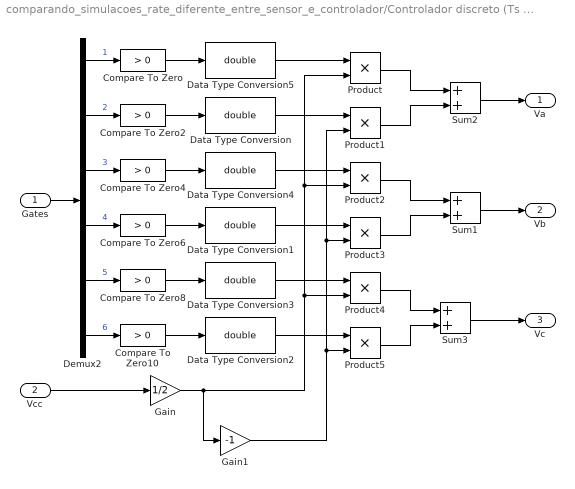
== system comparando_simulacoes_rate_diferente_entre_sensor_e_controlador/Controlador discreto (Ts = 0.001) Sensor discreto M (Ts = 0.01)/Inversor1 ==
  Gates : Inport
  Vcc : Inport  Port=2
  Compare To Zero : simulink/Logic and Bit Operations/Compare To Zero  relop=>  OutDataTypeStr=uint8  ZeroCross=off
  Compare To Zero{2,6,8,10} (4 alike) : simulink/Logic and Bit Operations/Compare To Zero  relop=>  OutDataTypeStr=boolean  ZeroCross=off
  Compare To Zero4 : simulink/Logic and Bit Operations/Compare To Zero  relop=>  OutDataTypeStr=uint8  ZeroCross=off
  Data Type Conversion{,1..5} (6 alike) : DataTypeConversion  OutDataTypeStr=double
  Demux2 : Demux  Outputs=6
  Gain : Gain  Gain=1/2
  Gain1 : Gain  Gain=-1
  Product{,1..5} (6 alike) : Product  RndMeth=Zero
  Sum1 : Sum  SaturateOnIntegerOverflow=on
  Sum2 : Sum  SaturateOnIntegerOverflow=on
  Sum3 : Sum  SaturateOnIntegerOverflow=on
  Va : Outport
  Vb : Outport  Port=2
  Vc : Outport  Port=3
  wires:
  Gain/1 -> Product/2, Product2/2, Product4/2, Gain1/1
  Gain1/1 -> Product1/2, Product3/2, Product5/2
  Data Type Conversion5/1 -> Product/1
  Data Type Conversion/1 -> Product1/1
  Data Type Conversion4/1 -> Product2/1
  Data Type Conversion1/1 -> Product3/1
  Data Type Conversion3/1 -> Product4/1
  Data Type Conversion2/1 -> Product5/1
  Product5/1 -> Sum3/2
  Product4/1 -> Sum3/1
  Product3/1 -> Sum1/2
  Product2/1 -> Sum1/1
  Product1/1 -> Sum2/2
  Product/1 -> Sum2/1
  Compare To Zero10/1 -> Data Type Conversion2/1
  Compare To Zero8/1 -> Data Type Conversion3/1
  Compare To Zero6/1 -> Data Type Conversion1/1
  Compare To Zero4/1 -> Data Type Conversion4/1
  Compare To Zero2/1 -> Data Type Conversion/1
  Compare To Zero/1 -> Data Type Conversion5/1
  Demux2/6 -> Compare To Zero10/1  "6"
  Demux2/5 -> Compare To Zero8/1  "5"
  Demux2/4 -> Compare To Zero6/1  "4"
  Demux2/3 -> Compare To Zero4/1  "3"
  Demux2/2 -> Compare To Zero2/1  "2"
  Demux2/1 -> Compare To Zero/1  "1"
  Gates/1 -> Demux2/1
  Sum2/1 -> Va/1
  Sum3/1 -> Vc/1
  Sum1/1 -> Vb/1
  Vcc/1 -> Gain/1

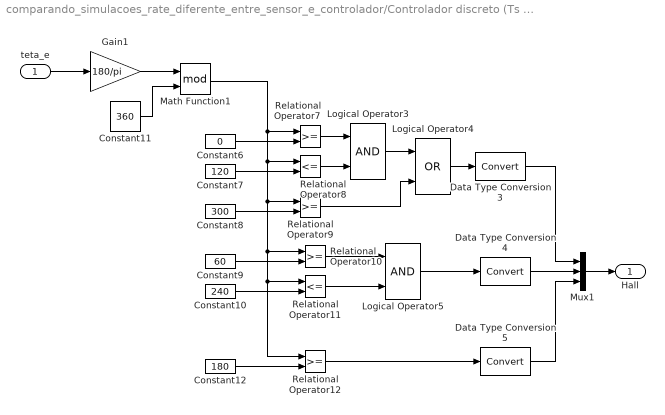
== system comparando_simulacoes_rate_diferente_entre_sensor_e_controlador/Controlador discreto (Ts = 0.001) Sensor discreto M (Ts = 0.01)/Sensores Hall1 ==
  teta_e : Inport
  Constant10 : Constant  Value=240
  Constant11 : Constant  Value=360
  Constant12 : Constant  Value=180
  Constant6 : Constant  Value=0
  Constant7 : Constant  Value=120
  Constant8 : Constant  Value=300
  Constant9 : Constant  Value=60
  Data Type Conversion3 : DataTypeConversion  SaturateOnIntegerOverflow=on  RndMeth=Zero
  Data Type Conversion4 : DataTypeConversion  SaturateOnIntegerOverflow=on  RndMeth=Zero
  Data Type Conversion5 : DataTypeConversion  SaturateOnIntegerOverflow=on  RndMeth=Zero
  Gain1 : Gain  Gain=180/pi
  Logical Operator3 : Logic  AllPortsSameDT=off  OutDataTypeStr=boolean
  Logical Operator4 : Logic  Operator=OR  AllPortsSameDT=off  OutDataTypeStr=boolean
  Logical Operator5 : Logic  AllPortsSameDT=off  OutDataTypeStr=boolean
  Math Function1 : Math  Operator=mod  SaturateOnIntegerOverflow=on
  Mux1 : Mux  Inputs=3
  Relational Operator{7,9..10,12} (4 alike) : RelationalOperator  InputSameDT=on
  Relational Operator11 : RelationalOperator  Operator=<=  InputSameDT=on
  Relational Operator8 : RelationalOperator  Operator=<=  InputSameDT=on
  Hall : Outport
  wires:
  Math Function1/1 -> Relational Operator7/1, Relational Operator12/1, Relational Operator11/1, Relational Operator10/1, Relational Operator9/1, Relational Operator8/1
  Constant11/1 -> Math Function1/2
  Gain1/1 -> Math Function1/1
  Relational Operator12/1 -> Data Type Conversion5/1
  Logical Operator5/1 -> Data Type Conversion4/1
  Logical Operator4/1 -> Data Type Conversion3/1
  Data Type Conversion5/1 -> Mux1/3
  Data Type Conversion4/1 -> Mux1/2
  Data Type Conversion3/1 -> Mux1/1
  Mux1/1 -> Hall/1
  Constant12/1 -> Relational Operator12/2
  Constant10/1 -> Relational Operator11/2
  Constant9/1 -> Relational Operator10/2
  Relational Operator11/1 -> Logical Operator5/2
  Relational Operator10/1 -> Logical Operator5/1
  Relational Operator8/1 -> Logical Operator3/2
  Relational Operator7/1 -> Logical Operator3/1
  Logical Operator3/1 -> Logical Operator4/1
  Relational Operator9/1 -> Logical Operator4/2
  Constant8/1 -> Relational Operator9/2
  Constant7/1 -> Relational Operator8/2
  Constant6/1 -> Relational Operator7/2
  teta_e/1 -> Gain1/1

== system comparando_simulacoes_rate_diferente_entre_sensor_e_controlador/Controlador discreto (Ts = 0.01) Sensor discreto M (Ts = 0.01)/BLDC1 ==
  Va : Inport
  Vb : Inport  Port=2
  Vc : Inport  Port=3
  Tl : Inport  Port=4
  "Cálculo Torque fase \"a\"" : Subsystem
  "Cálculo Torque fase \"b\"" : Subsystem
  "Cálculo Torque fase \"c\"" : Subsystem
  Cálculo das FCEMs : Subsystem
  "Dinâmica fase \"a\"" : Subsystem
  "Dinâmica fase \"b\"" : Subsystem
  "Dinâmica fase \"c\"" : Subsystem
  "Dinâmica mecânica " : Subsystem
  FCEMs : Scope  NumInputPorts=3
      settings: TimeRange=1  YMin=420~-5~-5  YMax=510~5~5  SaveName=ScopeData5
  Gain2 : Gain  Gain=P/2
  Scope : Scope
      settings: TimeRange=1  YMin=420  YMax=510  SaveName=ScopeData4
  Sum : Sum  Inputs=+++
  Vs : Scope  NumInputPorts=3
      settings: TimeRange=1  YMin=420~-5~-5  YMax=510~5~5  SaveName=ScopeData2
  is : Scope  NumInputPorts=3
      settings: TimeRange=1  YMin=420~-5~-5  YMax=510~5~5  SaveName=ScopeData3
  is1 : Scope  NumInputPorts=3
      settings: TimeRange=1  YMin=420~-5~-5  YMax=510~5~5  SaveName=ScopeData6
  Theta_m : Outport
  w_m : Outport  Port=2
  wires:
  Cálculo das FCEMs/1(e_a) -> FCEMs/1, "Dinâmica fase \"a\""/2(e_a)  "e_a"
  Cálculo das FCEMs/2(e_b) -> "Dinâmica fase \"b\""/2(e_b), FCEMs/2  "e_b"
  Cálculo das FCEMs/3(e_c) -> FCEMs/3, "Dinâmica fase \"c\""/2(e_c)  "e_c"
  Va/1 -> Vs/1, "Dinâmica fase \"a\""/1(Va)
  Vb/1 -> Vs/2, "Dinâmica fase \"b\""/1(Vb)
  Vc/1 -> Vs/3, "Dinâmica fase \"c\""/1(Vc)
  "Dinâmica fase \"a\""/1(i_a) -> is/1, "Cálculo Torque fase \"a\""/1(i_a)  "i_a"
  "Dinâmica fase \"b\""/1(i_b) -> is/2, "Cálculo Torque fase \"b\""/1(i_b)  "i_b"
  "Dinâmica fase \"c\""/1(i_c) -> is/3, "Cálculo Torque fase \"c\""/1(i_c)  "i_c"
  "Cálculo Torque fase \"a\""/1(T_a) -> is1/1, Sum/1  "T_a"
  "Cálculo Torque fase \"b\""/1(T_b) -> is1/2, Sum/2  "T_b"
  "Cálculo Torque fase \"c\""/1(T_c) -> is1/3, Sum/3  "T_c"
  Sum/1 -> Scope/1, "Dinâmica mecânica "/1(Te)  "T"
  "Dinâmica mecânica "/1(Theta_m) -> Theta_m/1, Gain2/1  "Theta_m"
  "Dinâmica mecânica "/2(w_m) -> Cálculo das FCEMs/2(w_m), w_m/1  "w_m"
  Tl/1 -> "Dinâmica mecânica "/2(Tl)
  Gain2/1 -> "Cálculo Torque fase \"a\""/2(Theta_e), "Cálculo Torque fase \"c\""/2(Theta_e), Cálculo das FCEMs/1(Theta_e), "Cálculo Torque fase \"b\""/2(Theta_e)

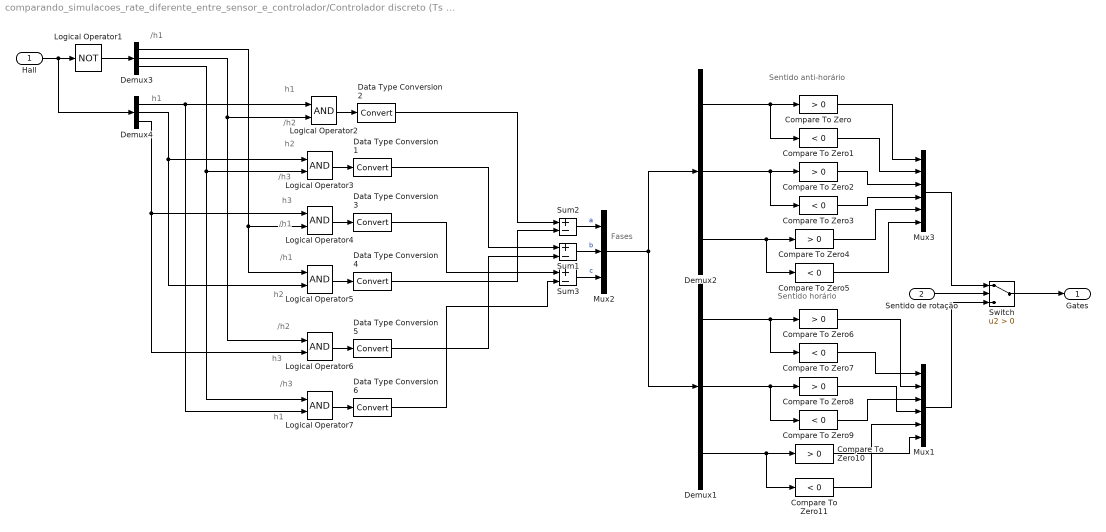
== system comparando_simulacoes_rate_diferente_entre_sensor_e_controlador/Controlador discreto (Ts = 0.01) Sensor discreto M (Ts = 0.01)/Decoder1 ==
  note: Fases
  note: Sentido horário
  note: Sentido anti-horário
  note: h1
  note: /h3
  note: h3
  note: /h2
  note: h2
  note: /h1
  note: /h1
  note: h3
  note: /h3
  note: h2
  note: /h2
  note: h1
  note: h1
  note: /h1
  "Hall " : Inport
  Sentido de rotação : Inport  Port=2
  Compare To Zero{,2,4,6,8,10} (6 alike) : simulink/Logic and Bit Operations/Compare To Zero  relop=>  OutDataTypeStr=boolean  ZeroCross=off
  Compare To Zero{1,3,5,7,9,11} (6 alike) : simulink/Logic and Bit Operations/Compare To Zero  relop=<  OutDataTypeStr=boolean  ZeroCross=off
  Data Type Conversion{1..6} (6 alike) : DataTypeConversion
  Demux{1..4} (4 alike) : Demux  Outputs=3
  Logical Operator1 : Logic  Operator=NOT  AllPortsSameDT=off  OutDataTypeStr=boolean
  Logical Operator{2..7} (6 alike) : Logic  AllPortsSameDT=off  OutDataTypeStr=boolean
  Mux1 : Mux  Inputs=6
  Mux2 : Mux  Inputs=3
  Mux3 : Mux  Inputs=6
  Sum1 : Sum  Inputs=+-  OutDataTypeStr=double
  Sum2 : Sum  Inputs=+-  OutDataTypeStr=double
  Sum3 : Sum  Inputs=+-  OutDataTypeStr=double
  Switch : Switch  Criteria=u2 > Threshold
  Gates : Outport
  wires:
  Mux2/1 -> Demux1/1, Demux2/1
  Data Type Conversion6/1 -> Sum3/2
  Data Type Conversion3/1 -> Sum3/1
  Data Type Conversion5/1 -> Sum1/2
  Data Type Conversion1/1 -> Sum1/1
  Data Type Conversion4/1 -> Sum2/2
  Data Type Conversion2/1 -> Sum2/1
  Logical Operator7/1 -> Data Type Conversion6/1
  Logical Operator6/1 -> Data Type Conversion5/1
  Logical Operator5/1 -> Data Type Conversion4/1
  Logical Operator4/1 -> Data Type Conversion3/1
  Logical Operator3/1 -> Data Type Conversion1/1
  Sum3/1 -> Mux2/3  "c"
  Sum1/1 -> Mux2/2  "b"
  Sum2/1 -> Mux2/1  "a"
  Logical Operator2/1 -> Data Type Conversion2/1
  Demux3/1 -> Logical Operator5/1, Logical Operator4/2
  Demux3/2 -> Logical Operator6/1, Logical Operator2/2
  Demux3/3 -> Logical Operator7/1, Logical Operator3/2
  Demux4/1 -> Logical Operator7/2, Logical Operator2/1
  Demux4/2 -> Logical Operator5/2, Logical Operator3/1
  Demux4/3 -> Logical Operator6/2, Logical Operator4/1
  Logical Operator1/1 -> Demux3/1
  "Hall "/1 -> Demux4/1, Logical Operator1/1
  Compare To Zero10/1 -> Mux1/6
  Compare To Zero11/1 -> Mux1/5
  Compare To Zero8/1 -> Mux1/4
  Compare To Zero9/1 -> Mux1/3
  Compare To Zero6/1 -> Mux1/2
  Compare To Zero7/1 -> Mux1/1
  Switch/1 -> Gates/1
  Mux1/1 -> Switch/3
  Sentido de rotação/1 -> Switch/2
  Mux3/1 -> Switch/1
  Demux1/3 -> Compare To Zero11/1, Compare To Zero10/1
  Demux1/2 -> Compare To Zero9/1, Compare To Zero8/1
  Demux1/1 -> Compare To Zero7/1, Compare To Zero6/1
  Compare To Zero5/1 -> Mux3/6
  Compare To Zero4/1 -> Mux3/5
  Compare To Zero3/1 -> Mux3/4
  Compare To Zero2/1 -> Mux3/3
  Compare To Zero1/1 -> Mux3/2
  Compare To Zero/1 -> Mux3/1
  Demux2/3 -> Compare To Zero5/1, Compare To Zero4/1
  Demux2/2 -> Compare To Zero3/1, Compare To Zero2/1
  Demux2/1 -> Compare To Zero1/1, Compare To Zero/1

== system comparando_simulacoes_rate_diferente_entre_sensor_e_controlador/Controlador discreto (Ts = 0.01) Sensor discreto M (Ts = 0.01)/Encoder ==
  note: ATENÇÃO: Para o correto funcionamento desse encoder o step size da simulação deve ser menor do que 360/(4*Nr*Vmax),
      | onde Vmax é o valor máximo da derivada do Theta atigindo durante a simulação
  Theta : Inport
  Determinar direçao : Subsystem
  Graus / pulso1 : Gain  Gain=360/(4*Nr)  OutDataTypeStr=double
  Método M : Subsystem  mask{Ts=0.01}
      mask prompts: Ts "Sampling time"
  Método T : Subsystem  mask{m=1}
      mask prompts: m "Número de pulsos que o bloco espera para calcular a velocidade média"
  Sensor Óptico : Subsystem
  Sensor Óptico1 : Subsystem
  Subsystem : Subsystem
  Theta_amostrado : Outport
  VelocidadeT : Outport  Port=2
  VelocidadeM : Outport  Port=3
  wires:
  Método M/1(Velocidade) -> VelocidadeM/1
  Método T/1(Velocidade) -> VelocidadeT/1
  Theta/1 -> Sensor Óptico/1(Theta), Sensor Óptico1/1(Theta)
  Graus / pulso1/1 -> Theta_amostrado/1, Método M/1(Posição)
  Subsystem/1(Out) -> Graus / pulso1/1
  Determinar direçao/2(NEG) -> Subsystem/2(NEG)
  Determinar direçao/1(POS) -> Subsystem/1(POS)
  Sensor Óptico1/1(Sinal_Pulso) -> Determinar direçao/2(B), Método T/2(B)  "B"
  Sensor Óptico/1(Sinal_Pulso) -> Método T/1(A), Determinar direçao/1(A)  "A"

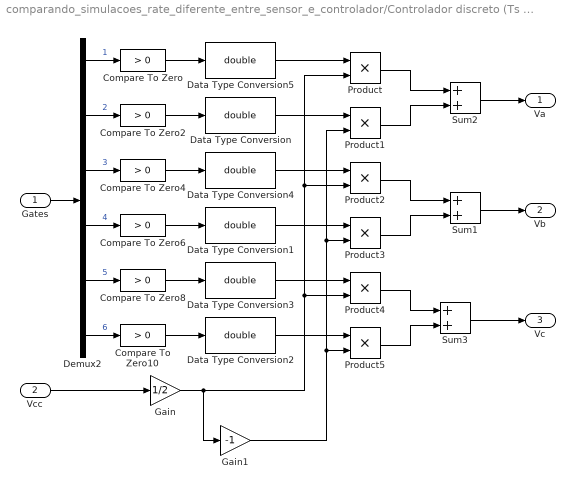
== system comparando_simulacoes_rate_diferente_entre_sensor_e_controlador/Controlador discreto (Ts = 0.01) Sensor discreto M (Ts = 0.01)/Inversor1 ==
  Gates : Inport
  Vcc : Inport  Port=2
  Compare To Zero : simulink/Logic and Bit Operations/Compare To Zero  relop=>  OutDataTypeStr=uint8  ZeroCross=off
  Compare To Zero{2,6,8,10} (4 alike) : simulink/Logic and Bit Operations/Compare To Zero  relop=>  OutDataTypeStr=boolean  ZeroCross=off
  Compare To Zero4 : simulink/Logic and Bit Operations/Compare To Zero  relop=>  OutDataTypeStr=uint8  ZeroCross=off
  Data Type Conversion{,1..5} (6 alike) : DataTypeConversion  OutDataTypeStr=double
  Demux2 : Demux  Outputs=6
  Gain : Gain  Gain=1/2
  Gain1 : Gain  Gain=-1
  Product{,1..5} (6 alike) : Product  RndMeth=Zero
  Sum1 : Sum  SaturateOnIntegerOverflow=on
  Sum2 : Sum  SaturateOnIntegerOverflow=on
  Sum3 : Sum  SaturateOnIntegerOverflow=on
  Va : Outport
  Vb : Outport  Port=2
  Vc : Outport  Port=3
  wires:
  Vcc/1 -> Gain/1
  Sum1/1 -> Vb/1
  Sum3/1 -> Vc/1
  Sum2/1 -> Va/1
  Gates/1 -> Demux2/1
  Demux2/1 -> Compare To Zero/1  "1"
  Demux2/2 -> Compare To Zero2/1  "2"
  Demux2/3 -> Compare To Zero4/1  "3"
  Demux2/4 -> Compare To Zero6/1  "4"
  Demux2/5 -> Compare To Zero8/1  "5"
  Demux2/6 -> Compare To Zero10/1  "6"
  Compare To Zero/1 -> Data Type Conversion5/1
  Compare To Zero2/1 -> Data Type Conversion/1
  Compare To Zero4/1 -> Data Type Conversion4/1
  Compare To Zero6/1 -> Data Type Conversion1/1
  Compare To Zero8/1 -> Data Type Conversion3/1
  Compare To Zero10/1 -> Data Type Conversion2/1
  Product/1 -> Sum2/1
  Product1/1 -> Sum2/2
  Product2/1 -> Sum1/1
  Product3/1 -> Sum1/2
  Product4/1 -> Sum3/1
  Product5/1 -> Sum3/2
  Data Type Conversion2/1 -> Product5/1
  Data Type Conversion3/1 -> Product4/1
  Data Type Conversion1/1 -> Product3/1
  Data Type Conversion4/1 -> Product2/1
  Data Type Conversion/1 -> Product1/1
  Data Type Conversion5/1 -> Product/1
  Gain1/1 -> Product5/2, Product3/2, Product1/2
  Gain/1 -> Gain1/1, Product4/2, Product2/2, Product/2

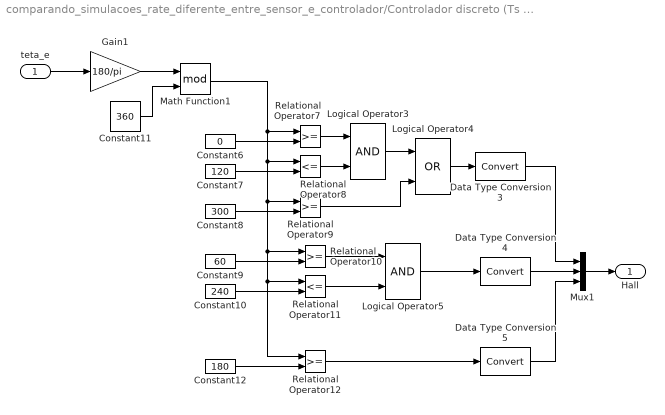
== system comparando_simulacoes_rate_diferente_entre_sensor_e_controlador/Controlador discreto (Ts = 0.01) Sensor discreto M (Ts = 0.01)/Sensores Hall1 ==
  teta_e : Inport
  Constant10 : Constant  Value=240
  Constant11 : Constant  Value=360
  Constant12 : Constant  Value=180
  Constant6 : Constant  Value=0
  Constant7 : Constant  Value=120
  Constant8 : Constant  Value=300
  Constant9 : Constant  Value=60
  Data Type Conversion3 : DataTypeConversion  SaturateOnIntegerOverflow=on  RndMeth=Zero
  Data Type Conversion4 : DataTypeConversion  SaturateOnIntegerOverflow=on  RndMeth=Zero
  Data Type Conversion5 : DataTypeConversion  SaturateOnIntegerOverflow=on  RndMeth=Zero
  Gain1 : Gain  Gain=180/pi
  Logical Operator3 : Logic  AllPortsSameDT=off  OutDataTypeStr=boolean
  Logical Operator4 : Logic  Operator=OR  AllPortsSameDT=off  OutDataTypeStr=boolean
  Logical Operator5 : Logic  AllPortsSameDT=off  OutDataTypeStr=boolean
  Math Function1 : Math  Operator=mod  SaturateOnIntegerOverflow=on
  Mux1 : Mux  Inputs=3
  Relational Operator{7,9..10,12} (4 alike) : RelationalOperator  InputSameDT=on
  Relational Operator11 : RelationalOperator  Operator=<=  InputSameDT=on
  Relational Operator8 : RelationalOperator  Operator=<=  InputSameDT=on
  Hall : Outport
  wires:
  teta_e/1 -> Gain1/1
  Constant6/1 -> Relational Operator7/2
  Constant7/1 -> Relational Operator8/2
  Constant8/1 -> Relational Operator9/2
  Relational Operator9/1 -> Logical Operator4/2
  Logical Operator3/1 -> Logical Operator4/1
  Relational Operator7/1 -> Logical Operator3/1
  Relational Operator8/1 -> Logical Operator3/2
  Relational Operator10/1 -> Logical Operator5/1
  Relational Operator11/1 -> Logical Operator5/2
  Constant9/1 -> Relational Operator10/2
  Constant10/1 -> Relational Operator11/2
  Constant12/1 -> Relational Operator12/2
  Mux1/1 -> Hall/1
  Data Type Conversion3/1 -> Mux1/1
  Data Type Conversion4/1 -> Mux1/2
  Data Type Conversion5/1 -> Mux1/3
  Logical Operator4/1 -> Data Type Conversion3/1
  Logical Operator5/1 -> Data Type Conversion4/1
  Relational Operator12/1 -> Data Type Conversion5/1
  Gain1/1 -> Math Function1/1
  Constant11/1 -> Math Function1/2
  Math Function1/1 -> Relational Operator8/1, Relational Operator9/1, Relational Operator10/1, Relational Operator11/1, Relational Operator12/1, Relational Operator7/1

== system comparando_simulacoes_rate_diferente_entre_sensor_e_controlador/Controle contínuo Sensor instantâneo/BLDC ==
  Va : Inport
  Vb : Inport  Port=2
  Vc : Inport  Port=3
  Tl : Inport  Port=4
  "Cálculo Torque fase \"a\"" : Subsystem
  "Cálculo Torque fase \"b\"" : Subsystem
  "Cálculo Torque fase \"c\"" : Subsystem
  Cálculo das FCEMs : Subsystem
  "Dinâmica fase \"a\"" : Subsystem
  "Dinâmica fase \"b\"" : Subsystem
  "Dinâmica fase \"c\"" : Subsystem
  "Dinâmica mecânica " : Subsystem
  FCEMs : Scope  NumInputPorts=3
      settings: TimeRange=1  YMin=420~-5~-5  YMax=510~5~5  SaveName=ScopeData5
  Gain2 : Gain  Gain=P/2
  Scope : Scope
      settings: TimeRange=1  YMin=420  YMax=510  SaveName=ScopeData4
  Sum : Sum  Inputs=+++
  Vs : Scope  NumInputPorts=3
      settings: TimeRange=1  YMin=420~-5~-5  YMax=510~5~5  SaveName=ScopeData2
  is : Scope  NumInputPorts=3
      settings: TimeRange=1  YMin=420~-5~-5  YMax=510~5~5  SaveName=ScopeData3
  is1 : Scope  NumInputPorts=3
      settings: TimeRange=1  YMin=420~-5~-5  YMax=510~5~5  SaveName=ScopeData6
  Theta_m : Outport
  w_m : Outport  Port=2
  wires:
  Cálculo das FCEMs/1(e_a) -> FCEMs/1, "Dinâmica fase \"a\""/2(e_a)  "e_a"
  Cálculo das FCEMs/2(e_b) -> "Dinâmica fase \"b\""/2(e_b), FCEMs/2  "e_b"
  Cálculo das FCEMs/3(e_c) -> FCEMs/3, "Dinâmica fase \"c\""/2(e_c)  "e_c"
  Va/1 -> Vs/1, "Dinâmica fase \"a\""/1(Va)
  Vb/1 -> Vs/2, "Dinâmica fase \"b\""/1(Vb)
  Vc/1 -> Vs/3, "Dinâmica fase \"c\""/1(Vc)
  "Dinâmica fase \"a\""/1(i_a) -> is/1, "Cálculo Torque fase \"a\""/1(i_a)  "i_a"
  "Dinâmica fase \"b\""/1(i_b) -> is/2, "Cálculo Torque fase \"b\""/1(i_b)  "i_b"
  "Dinâmica fase \"c\""/1(i_c) -> is/3, "Cálculo Torque fase \"c\""/1(i_c)  "i_c"
  "Cálculo Torque fase \"a\""/1(T_a) -> is1/1, Sum/1  "T_a"
  "Cálculo Torque fase \"b\""/1(T_b) -> is1/2, Sum/2  "T_b"
  "Cálculo Torque fase \"c\""/1(T_c) -> is1/3, Sum/3  "T_c"
  Sum/1 -> Scope/1, "Dinâmica mecânica "/1(Te)  "T"
  "Dinâmica mecânica "/1(Theta_m) -> Theta_m/1, Gain2/1  "Theta_m"
  "Dinâmica mecânica "/2(w_m) -> Cálculo das FCEMs/2(w_m), w_m/1  "w_m"
  Tl/1 -> "Dinâmica mecânica "/2(Tl)
  Gain2/1 -> "Cálculo Torque fase \"a\""/2(Theta_e), "Cálculo Torque fase \"c\""/2(Theta_e), Cálculo das FCEMs/1(Theta_e), "Cálculo Torque fase \"b\""/2(Theta_e)
